simulink model "dds_const_test"  (Simulink 7.0)
settings: Solver=VariableStepDiscrete  StartTime=0.0  StopTime=50  RelTol=1e-3
libraries: xbsIndex_r4 x9, casper_library x4
settings Model: Creator=User  LastModifiedBy=User
settings DebuggingCC: SaveWithDisabledLinksMsg=none  SaveWithParameterizedLinksMsg=none

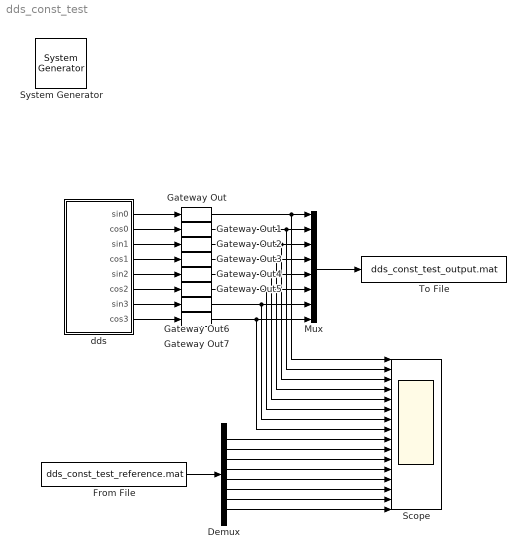
== system dds_const_test ==
  " System Generator" : xbsIndex_r4/ System Generator  Tag=genX  SystemSampleTime=-1  xilinxfamily=Virtex4  part=xc4vsx35  speed=-10  package=ff668  synthesis_tool=XST  clock_wrapper=Clock Enables  directory=./netlist  testbench=off  simulink_period=1  sysclk_period=100  dcm_input_clock_period=100  incr_netlist=off  trim_vbits=Everywhere in SubSystem  dbl_ovrd=According to Block Masks  core_generation=According to Block Masks  run_coregen=off  deprecated_control=off  eval_field=0  block_type=sysgen
      settings: block_version=10.1.1
  Demux : Demux  Outputs=8
  From File : FromFile  FileName=dds_const_test_reference.mat  SampleTime=1
  Gateway Out{,1..7} (8 alike) : xbsIndex_r4/Gateway Out  hdl_port=on  timing_constraint=None  locs_specified=off  LOCs={}  block_type=gatewayout
      settings: infoedit="Gateway out block.  Converts Xilinx fixed point inputs into ouputs of type Simulink integer, double, or fixed point.<P><P>Hardware notes:  In hardware these blocks become top level output ports or are discarded, depending on how they are configured."  block_version=10.1.1
  Mux : Mux  Inputs=8
  Scope : Scope  NumInputPorts=16
      settings: YMin=-5~-5~-5~-5~-5~-5~-5~-5~-5~-5~-5~-5~-5~-5~-5~-5  YMax=5~5~5~5~5~5~5~5~5~5~5~5~5~5~5~5
  To File : ToFile  Filename=dds_const_test_output.mat  MatrixName=output
  dds : Subsystem  AncestorBlock=casper_library/Downconverter/dds  mask(dds){freq_div=4, freq=2, num_lo=4, n_bits=10, latency=1}
      mask prompts: freq_div "Frequency divisions (M)"; freq "Frequency (? / M*2pi)"; num_lo "Parallel LOs"; n_bits "Bit Width"
      mask help:
      | Generates P channels of sin and cos data for mixing
      | with input data in a DDC. To generate frequency
      | N/M(Fc x P) (where Fc is the clock rate)
      | M = "Frequency Divisions", N = "Frequency",
      | Parallel LOs = P
      mask init:
      | dds_init(gcb, ...
      |     'freq_div', freq_div, ...
      |     'freq', freq, ...
      |     'num_lo', num_lo, ...
      |     'n_bits', n_bits, ...
      |     'latency', latency);
      settings: AttributesFormatString=lo at -2/4
      mask Help: eval('xlWeb([getenv(''MLIB_ROOT''), ''\doc\htmlblocks\sp_dds\sp_dds.html''])')
  wires:
  dds/1(sin0) -> Gateway Out/1
  dds/2(cos0) -> Gateway Out1/1
  dds/3(sin1) -> Gateway Out2/1
  dds/4(cos1) -> Gateway Out3/1
  Gateway Out/1 -> Mux/1, Scope/1
  Gateway Out1/1 -> Mux/2, Scope/2
  Gateway Out2/1 -> Mux/3, Scope/3
  Gateway Out3/1 -> Mux/4, Scope/4
  Mux/1 -> To File/1
  From File/1 -> Demux/1
  dds/5(sin2) -> Gateway Out4/1
  dds/6(cos2) -> Gateway Out5/1
  dds/7(sin3) -> Gateway Out6/1
  dds/8(cos3) -> Gateway Out7/1
  Gateway Out4/1 -> Mux/5, Scope/5
  Gateway Out5/1 -> Mux/6, Scope/6
  Gateway Out6/1 -> Mux/7, Scope/7
  Gateway Out7/1 -> Mux/8, Scope/8
  Demux/1 -> Scope/9
  Demux/2 -> Scope/10
  Demux/3 -> Scope/11
  Demux/4 -> Scope/12
  Demux/5 -> Scope/13
  Demux/6 -> Scope/14
  Demux/7 -> Scope/15
  Demux/8 -> Scope/16

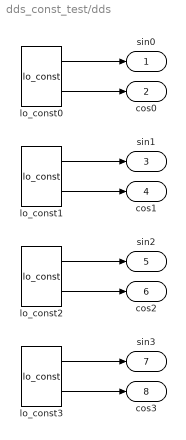
== system dds_const_test/dds ==
  lo_const0 : casper_library/Downconverter/lo_const  SystemSampleTime=-1  n_bits=10  phase=0
  lo_const1 : casper_library/Downconverter/lo_const  SystemSampleTime=-1  n_bits=10  phase=3.1416
  lo_const2 : casper_library/Downconverter/lo_const  SystemSampleTime=-1  n_bits=10  phase=6.2832
  lo_const3 : casper_library/Downconverter/lo_const  SystemSampleTime=-1  n_bits=10  phase=9.4248
  sin0 : Outport  OutDataType=sfix(16)  OutScaling=2^0
  cos0 : Outport  Port=2  OutDataType=sfix(16)  OutScaling=2^0
  sin1 : Outport  Port=3  OutDataType=sfix(16)  OutScaling=2^0
  cos1 : Outport  Port=4  OutDataType=sfix(16)  OutScaling=2^0
  sin2 : Outport  Port=5  OutDataType=sfix(16)  OutScaling=2^0
  cos2 : Outport  Port=6  OutDataType=sfix(16)  OutScaling=2^0
  sin3 : Outport  Port=7  OutDataType=sfix(16)  OutScaling=2^0
  cos3 : Outport  Port=8  OutDataType=sfix(16)  OutScaling=2^0
  wires:
  lo_const3/2 -> cos3/1
  lo_const3/1 -> sin3/1
  lo_const2/2 -> cos2/1
  lo_const2/1 -> sin2/1
  lo_const1/2 -> cos1/1
  lo_const1/1 -> sin1/1
  lo_const0/2 -> cos0/1
  lo_const0/1 -> sin0/1
